simulink model "system_identification_simulator"  (R2025b)
settings: Solver=VariableStepAuto  StartTime=0.0  StopTime=200  RelTol=1e-3
undefined symbols (not defined in the file or in its folder): MAP_model, paramGrecoMAP
settings Model: Creator=ciuba  LastModifiedBy=ciuba

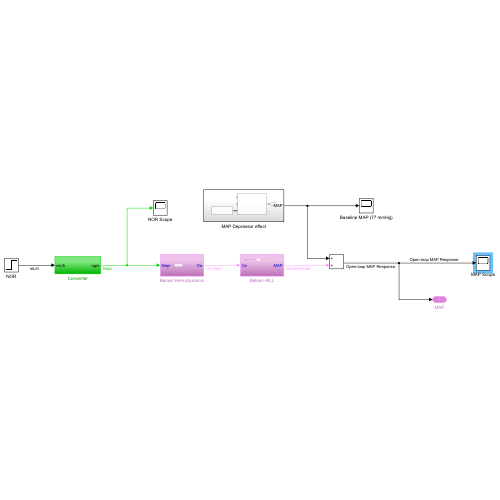
[thumbnail: Simulink's stored preview of the top-level diagram]
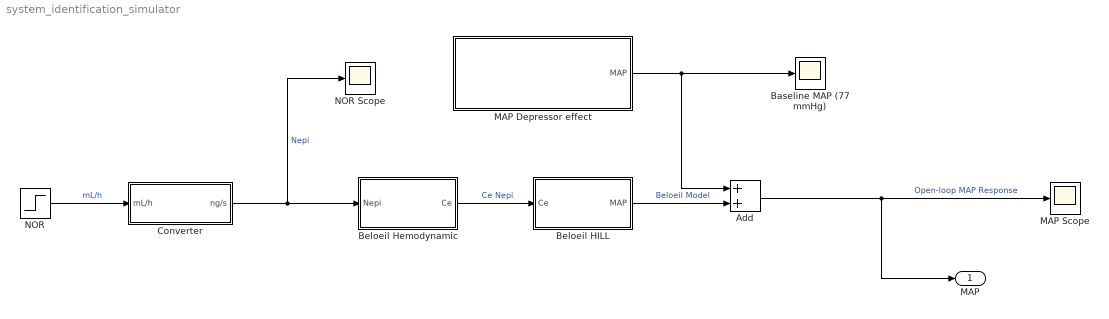
== system system_identification_simulator ==
  Add : Sum
  Baseline MAP (77 mmHg) : Scope
  Beloeil HILL : Subsystem
  Beloeil Hemodynamic : Subsystem
  Converter : Subsystem
  MAP Depressor effect : Subsystem
  MAP Scope : Scope
      settings: ActiveDisplayYMinimum=74.503233304108988  ActiveDisplayYMaximum=99.4709002630192  DataLoggingVariableName=ScopeData4
  NOR : Step  After=400  SampleTime=0
  NOR Scope : Scope
      settings: DataLoggingVariableName=ScopeData10  DataLoggingSaveFormat=Array
  MAP : Outport
  wires:
  Add/1 -> MAP/1, MAP Scope/1  "Open-loop MAP Response"
  MAP Depressor effect/1(MAP) -> Baseline MAP (77 mmHg)/1, Add/1
  Beloeil Hemodynamic/1(Ce) -> Beloeil HILL/1(Ce)  "Ce Nepi"
  NOR/1 -> Converter/1(mL/h)  "mL/h"
  Converter/1(ng/s) -> NOR Scope/1, Beloeil Hemodynamic/1(Nepi)  "Nepi"
  Beloeil HILL/1(MAP) -> Add/2  "Beloeil Model"

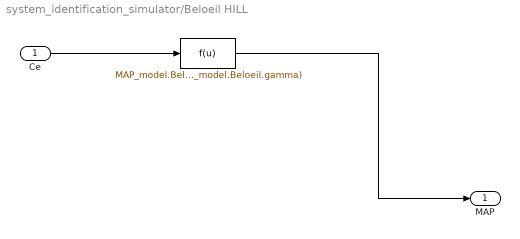
== system system_identification_simulator/Beloeil HILL ==
  Ce : Inport
  " " : Fcn  Expr=MAP_model.Beloeil.Emax * (u^MAP_model.Beloeil.gamma) / (MAP_model.Beloeil.EC50^MAP_model.Beloeil.gamma+u^MAP_model.Beloeil.gamma)
  MAP : Outport
  wires:
  " "/1 -> MAP/1
  Ce/1 -> " "/1

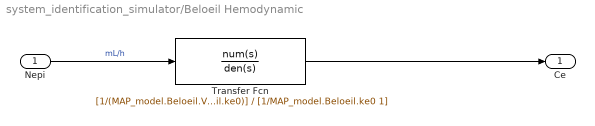
== system system_identification_simulator/Beloeil Hemodynamic ==
  Nepi : Inport
  Transfer Fcn : TransferFcn  Numerator=[1/(MAP_model.Beloeil.Vd*MAP_model.Beloeil.ke0)]  Denominator=[1/MAP_model.Beloeil.ke0 1]
  Ce : Outport
  wires:
  Nepi/1 -> Transfer Fcn/1  "mL/h"
  Transfer Fcn/1 -> Ce/1

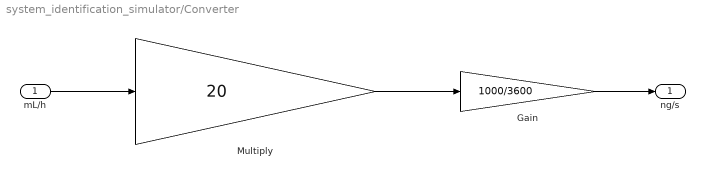
== system system_identification_simulator/Converter ==
  mL/h : Inport
  Gain : Gain  Gain=1000/3600
  Multiply : Gain  Gain=20
  ng/s : Outport
  wires:
  Gain/1 -> ng/s/1
  Multiply/1 -> Gain/1
  mL/h/1 -> Multiply/1

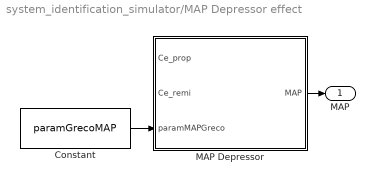
== system system_identification_simulator/MAP Depressor effect ==
  Constant : Constant  Value=paramGrecoMAP  OutDataTypeStr=Bus: GrecoMAPBus
  MAP Depressor : MATLAB Function  TreatAsAtomicUnit=on
  MAP : Outport
  wires:
  MAP Depressor/1(MAP) -> MAP/1
  Constant/1 -> MAP Depressor/3(paramMAPGreco)

== matlab function system_identification_simulator/MAP Depressor effect/MAP Depressor ==
  data: Ce_prop input; MAP output; Ce_remi input; paramMAPGreco input
function MAP = MAP_Greco(Ce_prop, Ce_remi, paramMAPGreco)    
    % Extract parameters from bus
    C50P   = paramMAPGreco.Prop.C50;    % Propofol EC50 (μg/mL)
    gammaP = paramMAPGreco.Prop.gamma;  % Propofol Hill
    C50R   = paramMAPGreco.Remi.C50;    % Remifentanil EC50 (ng/mL)
    gammaR = paramMAPGreco.Remi.gamma;  % Remifentanil Hill
    alpha  = paramMAPGreco.Interaction.alpha;  % Synergy parameter
    Emax   = paramMAPGreco.Interaction.Emax;   % Max MAP depression (mmHg)
    MAP0   = paramMAPGreco.Interaction.MAP0;   % Baseline MAP (mmHg)
    
    % Compute normalized concentrations
    X = (Ce_prop / C50P)^gammaP;
    Y = (Ce_remi / C50R)^gammaR;
    
    % Numerator/denominator as per Greco response surface
    numerator   = X + Y + alpha * X * Y;
    denominator = 1 + X + Y + alpha * X * Y;
    MAP_depr    = Emax * numerator / denominator;
    
    % Net MAP (subtract depressant effect from baseline)
    MAP = MAP0 - MAP_depr;
end
